simulink model "PR01_modelo"  (R2023a)
settings: Solver=FixedStepDiscrete  StartTime=0.0  StopTime=10.0  FixedStep=1  RelTol=1e-3
settings Model: Creator=santi  LastModifiedBy=santi

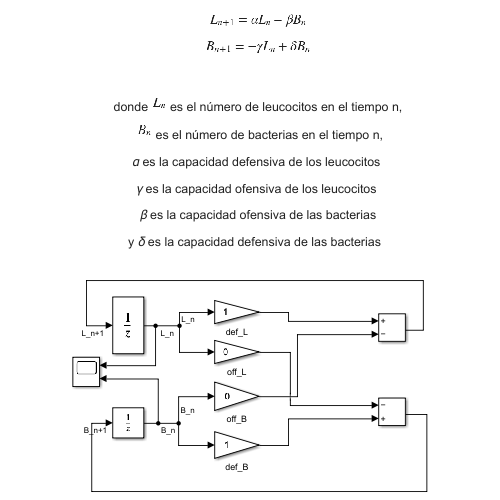
[thumbnail: Simulink's stored preview of the top-level diagram]
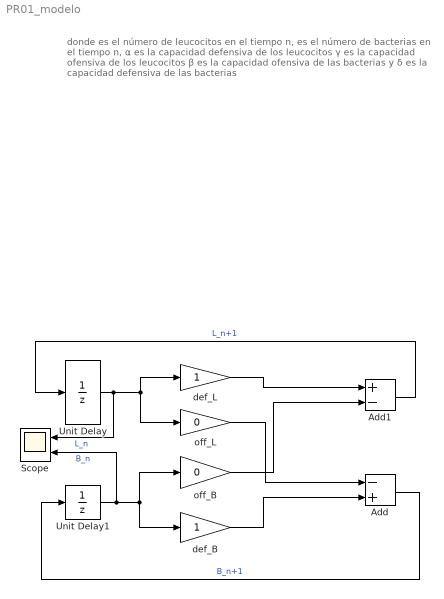
== system PR01_modelo ==
  note: donde es el número de leucocitos en el tiempo n,
      | es el número de bacterias en el tiempo n,
      | α es la capacidad defensiva de los leucocitos
      | γ es la capacidad ofensiva de los leucocitos
      | β es la capacidad ofensiva de las bacterias
      | y δ es la capacidad defensiva de las bacterias
  Add : Sum  Inputs=-+
  Add1 : Sum  Inputs=+-
  Scope : Scope  NumInputPorts=2
  Unit Delay : UnitDelay  InitialCondition=8000  SampleTime=-1  HasFrameUpgradeWarning=on
  Unit Delay1 : UnitDelay  InitialCondition=10000  SampleTime=-1  HasFrameUpgradeWarning=on
  def_B : Gain
  def_L : Gain
  off_B : Gain  Gain=0
  off_L : Gain  Gain=0
  wires:
  Unit Delay/1 -> Scope/1, off_L/1, def_L/1  "L_n"
  Add1/1 -> Unit Delay/1  "L_n+1"
  Unit Delay1/1 -> Scope/2, off_B/1, def_B/1  "B_n"
  Add/1 -> Unit Delay1/1  "B_n+1"
  off_L/1 -> Add/1
  def_B/1 -> Add/2
  def_L/1 -> Add1/1
  off_B/1 -> Add1/2
